simulink model "VehCtrlModl_autosar"  (R2019b)
settings: Solver=FixedStepDiscrete  StartTime=0.0  StopTime=10.0  RelTol=1e-3  EnableMultiTasking=on
settings Model: Creator=12045  LastModifiedBy=12045
settings SolverCC: AutoInsertRateTranBlk=on  InsertRTBMode=Never (minimum delay)
settings OptimizationCC: DefaultParameterBehavior=Inlined  EnhancedBackFolding=on  PassReuseOutputArgsAs=Individual arguments  ZeroExternalMemoryAtStartup=off  ZeroInternalMemoryAtStartup=off  OptimizeBlockOrder=speed  DifferentSizesBufferReuse=on  OptimizationCustomize=off  EfficientTunableParamExpr=on
settings DebuggingCC: MultiTaskDSMMsg=none  MultiTaskRateTransMsg=warning  ParameterTunabilityLossMsg=error  UnconnectedInputMsg=none  UnconnectedOutputMsg=none
settings SFSimCC: MATLABDynamicMemAlloc=off
settings RTWCC: Description=AUTOSAR  SystemTargetFile=autosar.tlc  GenCodeOnly=on  TemplateMakefile=ert_default_tmf  GenerateReport=on  IncludeHyperlinkInReport=on  LaunchReport=on  GenerateTraceInfo=on  GenerateTraceReport=on  GenerateTraceReportSl=on  GenerateTraceReportSf=on  GenerateTraceReportEml=on
settings CodeAppCC: ForceParamTrailComments=on  IgnoreCustomStorageClasses=off  OperatorAnnotations=on  SimulinkDataObjDesc=on  SFDataObjDesc=on  InsertBlockDesc=on
settings STFCustomTargetCC: TargetLangStandard=C99 (ISO)  MultiwordLength=256  ParMdlRefBuildCompliant=on  CompOptLevelCompliant=on  IncludeMdlTerminateFcn=off  CombineOutputUpdateFcns=on  SuppressErrorStatus=on  ERTCustomFileBanners=on  SupportNonFinite=off  SupportComplex=off  SupportContinuousTime=off  SupportNonInlinedSFcns=off  RemoveResetFunc=on  MATLABClassNameForMDSCustomization=Simulink.SoftwareTarget.ERTCustomization  AutosarCompliant=on  UseToolchainInfoCompliant=on  LookupTableObjectStructAxisOrder=2,1,3,4,...  LUTObjectStructOrderEvenSpacing=Size,Table,Breakpoints  SystemTargetFile=autosar.tlc
settings ERTTargetCC: TargetLangStandard=C99 (ISO)  ConcurrentExecutionCompliant=off  IncludeMdlTerminateFcn=off  SuppressErrorStatus=on  SupportNonFinite=off  SupportComplex=off  ModelStepFunctionPrototypeControlCompliant=off  CPPClassGenCompliant=off  AutosarCompliant=on  LookupTableObjectStructAxisOrder=2,1,3,4,...  LUTObjectStructOrderEvenSpacing=Size,Table,Breakpoints  InlinedParameterPlacement=NonHierarchical  ERTCustomFileTemplate=example_file_process.tlc

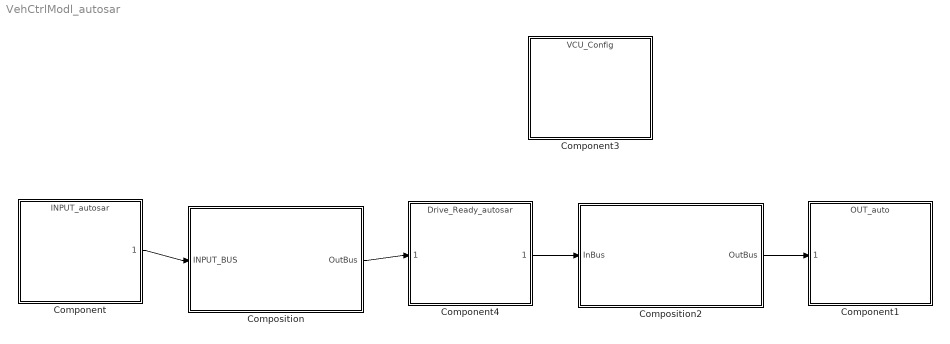
== system VehCtrlModl_autosar ==
  Component : ModelReference  ModelNameDialog=INPUT_autosar  SimulationMode=Normal  ScheduleRates=on  ScheduleRatesWith=Schedule Editor  ModelReferenceVersion=1.5
      settings: PortSchema="{\"entries\":[{\"content\":{\"headerSize\":38,\"margin\":15,\"minimumSpacing\":25,\"sides\":[{\"content\":{\"connectorIds\":[]},\"type\":\"ConnectorPlacement.EquallySpacedRectSide\",\"uuid\":\"3f144864-9d7e-4ef3-b53e-0b02a09b3f7c\"},{\"content\":{\"connectorIds\":[\"Out1\"],\"side\":\"RIGHT\"},\"type\":\"ConnectorPlacement.EquallySpacedRectSide\",\"uuid\":\"da086210-0760-4d07-8ae8-b6c94049e6d3\"},{\"content\":{\"connectorIds\":[],\"side\":\"TOP\"},\"type\":\"ConnectorPlacement.EquallySpacedRectSide\",\"uuid\":\"61bb60c6-ac1a-41d4-9e11-9f7d9465b8d9\"}]},\"type\":\"ConnectorPlacement.EquallySpacedConnector\",\"uuid\":\"6c6b6048-288a-4547-b024-c962ca493539\"}],\"packageUris\":[\"http://schema.mathworks.com/mf0/Connector/19700101\"],\"version\":\"1.0\"}"
  Component1 : ModelReference  ModelNameDialog=OUT_auto  SimulationMode=Normal  ScheduleRates=on  ScheduleRatesWith=Schedule Editor  ModelReferenceVersion=1.2
      settings: PortSchema="{\"entries\":[{\"content\":{\"headerSize\":38,\"margin\":15,\"minimumSpacing\":25,\"sides\":[{\"content\":{\"connectorIds\":[\"In1\"]},\"type\":\"ConnectorPlacement.EquallySpacedRectSide\",\"uuid\":\"972b8812-4f66-48e1-a50f-856a8ff4edf4\"},{\"content\":{\"connectorIds\":[],\"side\":\"RIGHT\"},\"type\":\"ConnectorPlacement.EquallySpacedRectSide\",\"uuid\":\"e79fdc99-55e6-49e3-9797-bdbb7463bac3\"},{\"content\":{\"connectorIds\":[],\"side\":\"TOP\"},\"type\":\"ConnectorPlacement.EquallySpacedRectSide\",\"uuid\":\"de5bfbcc-cc48-4777-a243-8708c691c562\"}]},\"type\":\"ConnectorPlacement.EquallySpacedConnector\",\"uuid\":\"f9db6440-ec3e-4ea2-95f6-630efa524718\"}],\"packageUris\":[\"http://schema.mathworks.com/mf0/Connector/19700101\"],\"version\":\"1.0\"}"
  Component3 : ModelReference  ModelNameDialog=VCU_Config  SimulationMode=Normal  ScheduleRates=on  ScheduleRatesWith=Schedule Editor  ModelReferenceVersion=1.5
      settings: PortSchema="{\"entries\":[{\"content\":{\"headerSize\":38,\"margin\":15,\"minimumSpacing\":25,\"sides\":[{\"content\":{\"connectorIds\":[]},\"type\":\"ConnectorPlacement.EquallySpacedRectSide\",\"uuid\":\"f43777d3-b52c-42ba-a281-f330c306dc52\"},{\"content\":{\"connectorIds\":[],\"side\":\"RIGHT\"},\"type\":\"ConnectorPlacement.EquallySpacedRectSide\",\"uuid\":\"3f6bc4af-72b0-4e1b-866b-b8109e033668\"},{\"content\":{\"connectorIds\":[],\"side\":\"TOP\"},\"type\":\"ConnectorPlacement.EquallySpacedRectSide\",\"uuid\":\"bc9ba6bb-8b91-41fc-b3ec-9308de82bedb\"}]},\"type\":\"ConnectorPlacement.EquallySpacedConnector\",\"uuid\":\"fee5ae7f-1a9c-43fd-b3cd-af0584f902f2\"}],\"packageUris\":[\"http://schema.mathworks.com/mf0/Connector/19700101\"],\"version\":\"1.0\"}"
  Component4 : ModelReference  ModelNameDialog=Drive_Ready_autosar  SimulationMode=Normal  ScheduleRates=on  ScheduleRatesWith=Schedule Editor  ModelReferenceVersion=1.4
      settings: PortSchema="{\"entries\":[{\"content\":{\"headerSize\":38,\"margin\":15,\"minimumSpacing\":25,\"sides\":[{\"content\":{\"connectorIds\":[\"In1\"]},\"type\":\"ConnectorPlacement.EquallySpacedRectSide\",\"uuid\":\"49d7a716-8d3c-407e-99f4-b11206eca66e\"},{\"content\":{\"connectorIds\":[\"Out1\"],\"side\":\"RIGHT\"},\"type\":\"ConnectorPlacement.EquallySpacedRectSide\",\"uuid\":\"4ef8d5bb-314e-40d0-9324-56f54f708f96\"},{\"content\":{\"connectorIds\":[],\"side\":\"TOP\"},\"type\":\"ConnectorPlacement.EquallySpacedRectSide\",\"uuid\":\"9f1a4d2b-3d6d-467b-a0e4-2ce29ab99e87\"}]},\"type\":\"ConnectorPlacement.EquallySpacedConnector\",\"uuid\":\"26a97e7b-8476-4a14-b139-2a926e7f2325\"}],\"packageUris\":[\"http://schema.mathworks.com/mf0/Connector/19700101\"],\"version\":\"1.0\"}"
  Composition : Subsystem
      settings: PortSchema="{\"entries\":[{\"content\":{\"headerSize\":26,\"margin\":15,\"minimumSpacing\":25,\"sides\":[{\"content\":{\"connectorIds\":[\"In1\"]},\"type\":\"ConnectorPlacement.EquallySpacedRectSide\",\"uuid\":\"49d7a716-8d3c-407e-99f4-b11206eca66e\"},{\"content\":{\"connectorIds\":[\"Out1\"],\"side\":\"RIGHT\"},\"type\":\"ConnectorPlacement.EquallySpacedRectSide\",\"uuid\":\"4ef8d5bb-314e-40d0-9324-56f54f708f96\"},{\"content\":{\"connectorIds\":[],\"side\":\"TOP\"},\"type\":\"ConnectorPlacement.EquallySpacedRectSide\",\"uuid\":\"9f1a4d2b-3d6d-467b-a0e4-2ce29ab99e87\"}]},\"type\":\"ConnectorPlacement.EquallySpacedConnector\",\"uuid\":\"26a97e7b-8476-4a14-b139-2a926e7f2325\"}],\"packageUris\":[\"http://schema.mathworks.com/mf0/Connector/19700101\"],\"version\":\"1.0\"}"
  Composition2 : Subsystem
      settings: PortSchema="{\"entries\":[{\"content\":{\"headerSize\":26,\"margin\":15,\"minimumSpacing\":25,\"sides\":[{\"content\":{\"connectorIds\":[\"In1\"]},\"type\":\"ConnectorPlacement.EquallySpacedRectSide\",\"uuid\":\"49d7a716-8d3c-407e-99f4-b11206eca66e\"},{\"content\":{\"connectorIds\":[\"Out1\"],\"side\":\"RIGHT\"},\"type\":\"ConnectorPlacement.EquallySpacedRectSide\",\"uuid\":\"4ef8d5bb-314e-40d0-9324-56f54f708f96\"},{\"content\":{\"connectorIds\":[],\"side\":\"TOP\"},\"type\":\"ConnectorPlacement.EquallySpacedRectSide\",\"uuid\":\"9f1a4d2b-3d6d-467b-a0e4-2ce29ab99e87\"}]},\"type\":\"ConnectorPlacement.EquallySpacedConnector\",\"uuid\":\"26a97e7b-8476-4a14-b139-2a926e7f2325\"}],\"packageUris\":[\"http://schema.mathworks.com/mf0/Connector/19700101\"],\"version\":\"1.0\"}"
  wires:
  Composition2/1(OutBus) -> Component1/1
  Component4/1 -> Composition2/1(InBus)
  Composition/1(OutBus) -> Component4/1
  Component/1 -> Composition/1(INPUT_BUS)

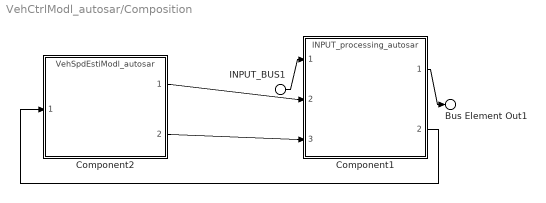
== system VehCtrlModl_autosar/Composition ==
  INPUT_BUS1 : Inport  PortName=INPUT_BUS
  Component1 : ModelReference  ModelNameDialog=INPUT_processing_autosar  SimulationMode=Normal  ScheduleRates=on  ScheduleRatesWith=Schedule Editor  ModelReferenceVersion=1.10
      settings: PortSchema="{\"entries\":[{\"content\":{\"headerSize\":38,\"margin\":15,\"minimumSpacing\":25,\"sides\":[{\"content\":{\"connectorIds\":[\"In1\",\"In2\",\"In3\"]},\"type\":\"ConnectorPlacement.EquallySpacedRectSide\",\"uuid\":\"3f144864-9d7e-4ef3-b53e-0b02a09b3f7c\"},{\"content\":{\"connectorIds\":[\"Out1\",\"Out2\"],\"side\":\"RIGHT\"},\"type\":\"ConnectorPlacement.EquallySpacedRectSide\",\"uuid\":\"da086210-0760-4d07-8ae8-b6c94049e6d3\"},{\"content\":{\"connectorIds\":[],\"side\":\"TOP\"},\"type\":\"ConnectorPlacement.EquallySpacedRectSide\",\"uuid\":\"61bb60c6-ac1a-41d4-9e11-9f7d9465b8d9\"}]},\"type\":\"ConnectorPlacement.EquallySpacedConnector\",\"uuid\":\"6c6b6048-288a-4547-b024-c962ca493539\"}],\"packageUris\":[\"http://schema.mathworks.com/mf0/Connector/19700101\"],\"version\":\"1.0\"}"
  Component2 : ModelReference  ModelNameDialog=VehSpdEstiModl_autosar  SimulationMode=Normal  ScheduleRates=on  ScheduleRatesWith=Schedule Editor  ModelReferenceVersion=1.5
      settings: PortSchema="{\"entries\":[{\"content\":{\"headerSize\":38,\"margin\":15,\"minimumSpacing\":25,\"sides\":[{\"content\":{\"connectorIds\":[\"In1\"]},\"type\":\"ConnectorPlacement.EquallySpacedRectSide\",\"uuid\":\"3f144864-9d7e-4ef3-b53e-0b02a09b3f7c\"},{\"content\":{\"connectorIds\":[\"Out1\",\"Out2\"],\"side\":\"RIGHT\"},\"type\":\"ConnectorPlacement.EquallySpacedRectSide\",\"uuid\":\"da086210-0760-4d07-8ae8-b6c94049e6d3\"},{\"content\":{\"connectorIds\":[],\"side\":\"TOP\"},\"type\":\"ConnectorPlacement.EquallySpacedRectSide\",\"uuid\":\"61bb60c6-ac1a-41d4-9e11-9f7d9465b8d9\"}]},\"type\":\"ConnectorPlacement.EquallySpacedConnector\",\"uuid\":\"6c6b6048-288a-4547-b024-c962ca493539\"}],\"packageUris\":[\"http://schema.mathworks.com/mf0/Connector/19700101\"],\"version\":\"1.0\"}"
  Bus Element Out1 : Outport  PortName=OutBus
  wires:
  Component1/1 -> Bus Element Out1/1
  Component2/2 -> Component1/3
  Component1/2 -> Component2/1
  Component2/1 -> Component1/2
  INPUT_BUS1/1 -> Component1/1

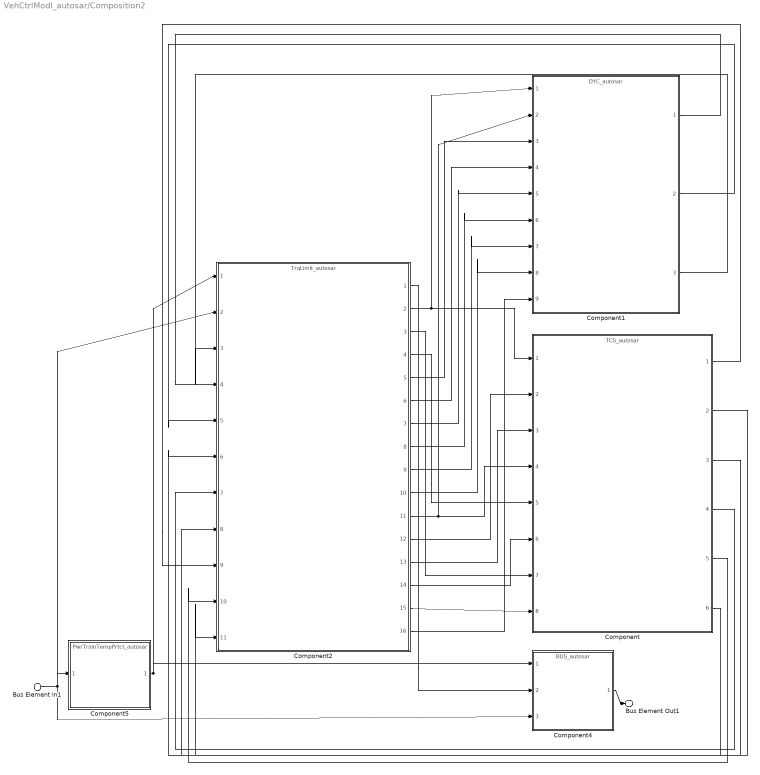
== system VehCtrlModl_autosar/Composition2 ==
  Bus Element In1 : Inport  PortName=InBus
  Component : ModelReference  ModelNameDialog=TCS_autosar  SimulationMode=Normal  ScheduleRates=on  ScheduleRatesWith=Schedule Editor  ModelReferenceVersion=1.7
      settings: PortSchema="{\"entries\":[{\"content\":{\"headerSize\":38,\"margin\":15,\"minimumSpacing\":25,\"sides\":[{\"content\":{\"connectorIds\":[\"In1\",\"In2\",\"In3\",\"In4\",\"In5\",\"In6\",\"In7\",\"In8\"]},\"type\":\"ConnectorPlacement.EquallySpacedRectSide\",\"uuid\":\"49d7a716-8d3c-407e-99f4-b11206eca66e\"},{\"content\":{\"connectorIds\":[\"Out1\",\"Out2\",\"Out3\",\"Out4\",\"Out5\",\"Out6\"],\"side\":\"RIGHT\"},\"type\":\"ConnectorPlacement.EquallySpacedRectSide\",\"uuid\":\"4ef8d5bb-314e-40d0-9324-56f54f708f96\"},{\"content\":{\"connectorIds\":[],\"side\":\"TOP\"},\"type\":\"ConnectorPlacement.EquallySpacedRectSide\",\"uuid\":\"9f1a4d2b-3d6d-467b-a0e4-2ce29ab99e87\"}]},\"type\":\"ConnectorPlacement.EquallySpacedConnector\",\"uuid\":\"26a97e7b-8476-4a14-b139-2a926e7f2325\"}],\"packageUris\":[\"http://schema.mathworks.com/mf0/Connector/19700101\"],\"version\":\"1.0\"}"
  Component1 : ModelReference  ModelNameDialog=DYC_autosar  SimulationMode=Normal  ScheduleRates=on  ScheduleRatesWith=Schedule Editor  ModelReferenceVersion=1.3
      settings: PortSchema="{\"entries\":[{\"content\":{\"headerSize\":38,\"margin\":15,\"minimumSpacing\":25,\"sides\":[{\"content\":{\"connectorIds\":[\"In1\",\"In2\",\"In3\",\"In4\",\"In5\",\"In6\",\"In7\",\"In8\",\"In9\"]},\"type\":\"ConnectorPlacement.EquallySpacedRectSide\",\"uuid\":\"49d7a716-8d3c-407e-99f4-b11206eca66e\"},{\"content\":{\"connectorIds\":[\"Out1\",\"Out2\",\"Out3\"],\"side\":\"RIGHT\"},\"type\":\"ConnectorPlacement.EquallySpacedRectSide\",\"uuid\":\"4ef8d5bb-314e-40d0-9324-56f54f708f96\"},{\"content\":{\"connectorIds\":[],\"side\":\"TOP\"},\"type\":\"ConnectorPlacement.EquallySpacedRectSide\",\"uuid\":\"9f1a4d2b-3d6d-467b-a0e4-2ce29ab99e87\"}]},\"type\":\"ConnectorPlacement.EquallySpacedConnector\",\"uuid\":\"26a97e7b-8476-4a14-b139-2a926e7f2325\"}],\"packageUris\":[\"http://schema.mathworks.com/mf0/Connector/19700101\"],\"version\":\"1.0\"}"
  Component2 : ModelReference  ModelNameDialog=TrqLimit_autosar  SimulationMode=Normal  ScheduleRates=on  ScheduleRatesWith=Schedule Editor  ModelReferenceVersion=1.8
      settings: PortSchema="{\"entries\":[{\"content\":{\"headerSize\":38,\"margin\":15,\"minimumSpacing\":25,\"sides\":[{\"content\":{\"connectorIds\":[\"In1\",\"In2\",\"In3\",\"In4\",\"In5\",\"In6\",\"In7\",\"In8\",\"In9\",\"In10\",\"In11\"]},\"type\":\"ConnectorPlacement.EquallySpacedRectSide\",\"uuid\":\"49d7a716-8d3c-407e-99f4-b11206eca66e\"},{\"content\":{\"connectorIds\":[\"Out1\",\"Out2\",\"Out3\",\"Out4\",\"Out5\",\"Out6\",\"Out7\",\"Out8\",\"Out9\",\"Out10\",\"Out11\",\"Out12\",\"Out13\",\"Out14\",\"Out15\",\"Out16\"],\"side\":\"RIGHT\"},\"type\":\"ConnectorPlacement.EquallySpacedRectSide\",\"uuid\":\"4ef8d5bb-314e-40d0-9324-56f54f708f96\"},{\"content\":{\"connectorIds\":[],\"side\":\"TOP\"},\"type\":\"ConnectorPlacement.EquallySpacedRectSide\",\"uuid\":\"9f1a4d2b-3d6d-467b-a0e4-2ce29ab99e87\"}]},\"type\":\"ConnectorPlacement.EquallySpacedConnector\",\"uuid\":\"26a97e7b-8476-4a14-b139-2a926e7f2325\"}],\"packageUris\":[\"http://schema.mathworks.com/mf0/Connector/19700101\"],\"version\":\"1.0\"}"
  Component4 : ModelReference  ModelNameDialog=BUS_autosar  SimulationMode=Normal  ScheduleRates=on  ScheduleRatesWith=Schedule Editor  ModelReferenceVersion=1.2
      settings: PortSchema="{\"entries\":[{\"content\":{\"headerSize\":38,\"margin\":15,\"minimumSpacing\":25,\"sides\":[{\"content\":{\"connectorIds\":[\"In1\",\"In2\",\"In3\"]},\"type\":\"ConnectorPlacement.EquallySpacedRectSide\",\"uuid\":\"972b8812-4f66-48e1-a50f-856a8ff4edf4\"},{\"content\":{\"connectorIds\":[\"Out1\"],\"side\":\"RIGHT\"},\"type\":\"ConnectorPlacement.EquallySpacedRectSide\",\"uuid\":\"e79fdc99-55e6-49e3-9797-bdbb7463bac3\"},{\"content\":{\"connectorIds\":[],\"side\":\"TOP\"},\"type\":\"ConnectorPlacement.EquallySpacedRectSide\",\"uuid\":\"de5bfbcc-cc48-4777-a243-8708c691c562\"}]},\"type\":\"ConnectorPlacement.EquallySpacedConnector\",\"uuid\":\"f9db6440-ec3e-4ea2-95f6-630efa524718\"}],\"packageUris\":[\"http://schema.mathworks.com/mf0/Connector/19700101\"],\"version\":\"1.0\"}"
  Component5 : ModelReference  ModelNameDialog=PwrTrainTempPrtct_autosar  SimulationMode=Normal  ScheduleRates=on  ScheduleRatesWith=Schedule Editor  ModelReferenceVersion=1.4
      settings: PortSchema="{\"entries\":[{\"content\":{\"headerSize\":38,\"margin\":15,\"minimumSpacing\":25,\"sides\":[{\"content\":{\"connectorIds\":[\"In1\"]},\"type\":\"ConnectorPlacement.EquallySpacedRectSide\",\"uuid\":\"49d7a716-8d3c-407e-99f4-b11206eca66e\"},{\"content\":{\"connectorIds\":[\"Out1\"],\"side\":\"RIGHT\"},\"type\":\"ConnectorPlacement.EquallySpacedRectSide\",\"uuid\":\"4ef8d5bb-314e-40d0-9324-56f54f708f96\"},{\"content\":{\"connectorIds\":[],\"side\":\"TOP\"},\"type\":\"ConnectorPlacement.EquallySpacedRectSide\",\"uuid\":\"9f1a4d2b-3d6d-467b-a0e4-2ce29ab99e87\"}]},\"type\":\"ConnectorPlacement.EquallySpacedConnector\",\"uuid\":\"26a97e7b-8476-4a14-b139-2a926e7f2325\"}],\"packageUris\":[\"http://schema.mathworks.com/mf0/Connector/19700101\"],\"version\":\"1.0\"}"
  Bus Element Out1 : Outport  PortName=OutBus
  wires:
  Component2/11 -> Component1/2, Component/4
  Component5/1 -> Component2/1, Component4/1
  Component2/16 -> Component1/9
  Component2/1 -> Component4/2
  Component/3 -> Component2/11
  Component/1 -> Component2/9
  Component/5 -> Component2/10
  Component/4 -> Component2/7
  Component/2 -> Component2/6
  Component2/15 -> Component/8
  Component2/8 -> Component1/6
  Component2/14 -> Component/6
  Component2/7 -> Component1/5
  Component2/13 -> Component/3
  Component2/9 -> Component1/7
  Component2/6 -> Component1/4
  Component/6 -> Component2/8
  Component2/5 -> Component1/3
  Component1/1 -> Component2/4
  Component2/2 -> Component1/1, Component/1
  Component1/2 -> Component2/5
  Component1/3 -> Component2/3
  Component2/10 -> Component1/8
  Component2/12 -> Component/2
  Component2/3 -> Component/7
  Component2/4 -> Component/5
  Bus Element In1/1 -> Component2/2, Component5/1, Component4/3
  Component4/1 -> Bus Element Out1/1
